simulink model "untitled"  (R2016a)
settings: Solver=VariableStepAuto  StartTime=0.0  StopTime=10.0  RelTol=1e-3
libraries: simulink x1
settings Model: Creator=wojta  LastModifiedBy=wojta

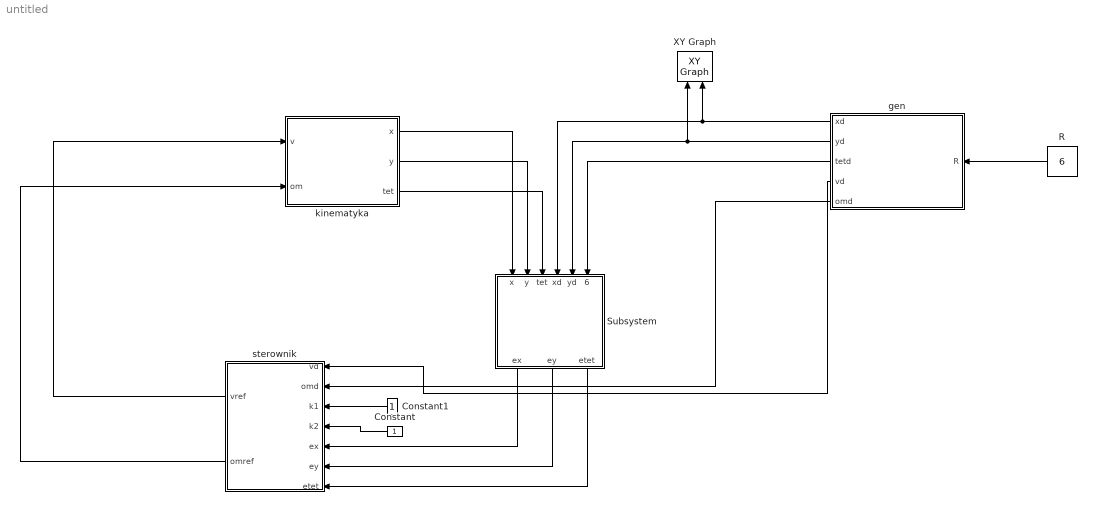
== system untitled ==
  Constant : Constant
  Constant1 : Constant
  R : Constant  Value=6
  Subsystem : Subsystem
  XY Graph : simulink/Sinks/XY Graph  xmin=-6  xmax=6  ymin=-6  ymax=6  st=-1
  gen : Subsystem
  kinematyka : Subsystem
  sterownik : Subsystem
  wires:
  R/1 -> gen/1(R)
  sterownik/1(vref) -> kinematyka/1(v)
  sterownik/2(omref) -> kinematyka/2(om)
  kinematyka/1(x) -> Subsystem/1(x)
  kinematyka/2(y) -> Subsystem/2(y)
  kinematyka/3(tet) -> Subsystem/3(tet)
  gen/1(xd) -> XY Graph/2, Subsystem/4(xd)
  gen/2(yd) -> XY Graph/1, Subsystem/5(yd)
  gen/3(tetd) -> Subsystem/6(tetd)
  Subsystem/1(ex) -> sterownik/5(ex)
  Subsystem/2(ey) -> sterownik/6(ey)
  Subsystem/3(etet) -> sterownik/7(etet)
  gen/4(vd) -> sterownik/1(vd)
  gen/5(omd) -> sterownik/2(omd)
  Constant1/1 -> sterownik/3(k1)
  Constant/1 -> sterownik/4(k2)

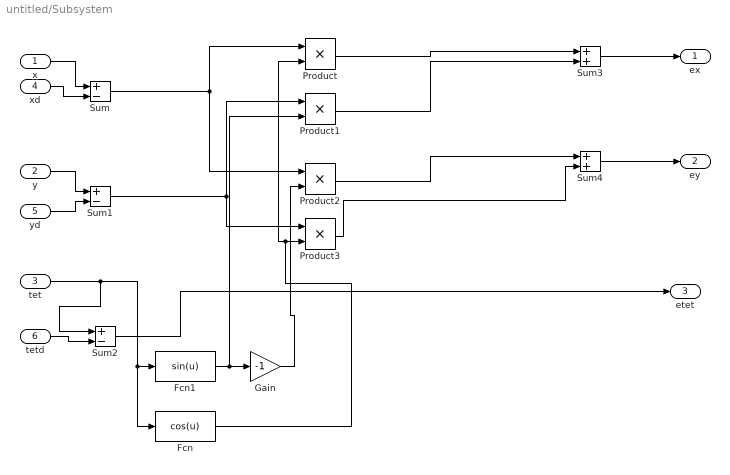
== system untitled/Subsystem ==
  x : Inport
  y : Inport  Port=2
  tet : Inport  Port=3
  xd : Inport  Port=4
  yd : Inport  Port=5
  tetd : Inport  Port=6
  Fcn : Fcn  Expr=cos(u)
  Fcn1 : Fcn  Expr=sin(u)
  Gain : Gain  Gain=-1
  Product{,1..3} (4 alike) : Product
  Sum : Sum  Inputs=+-
  Sum1 : Sum  Inputs=+-
  Sum2 : Sum  Inputs=+-
  Sum3 : Sum
  Sum4 : Sum
  ex : Outport
  ey : Outport  Port=2
  etet : Outport  Port=3
  wires:
  xd/1 -> Sum/2
  yd/1 -> Sum1/2
  Product3/1 -> Sum4/2
  tetd/1 -> Sum2/2
  Fcn1/1 -> Product1/2, Gain/1
  Product1/1 -> Sum3/2
  tet/1 -> Fcn/1, Fcn1/1, Sum2/1
  Gain/1 -> Product2/2
  Product2/1 -> Sum4/1
  Sum2/1 -> etet/1
  y/1 -> Sum1/1
  Product/1 -> Sum3/1
  Sum1/1 -> Product3/1, Product1/1
  Sum4/1 -> ey/1
  x/1 -> Sum/1
  Fcn/1 -> Product/2, Product3/2
  Sum3/1 -> ex/1
  Sum/1 -> Product/1, Product2/1

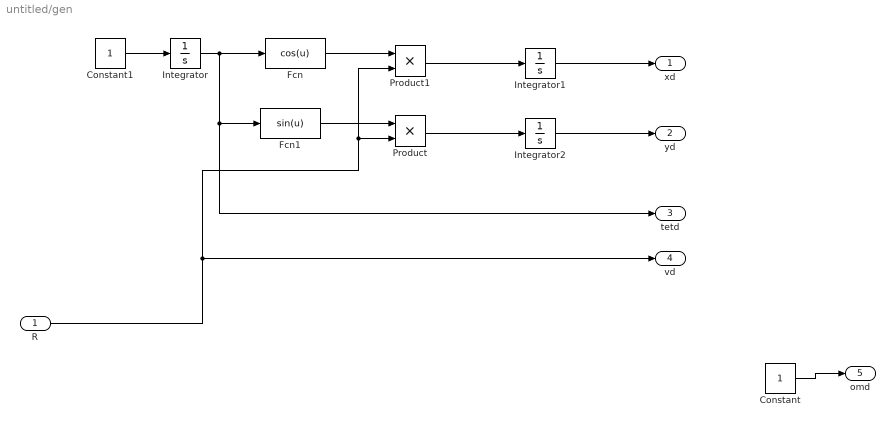
== system untitled/gen ==
  R : Inport
  Constant : Constant
  Constant1 : Constant
  Fcn : Fcn  Expr=cos(u)
  Fcn1 : Fcn  Expr=sin(u)
  Integrator : Integrator
  Integrator1 : Integrator
  Integrator2 : Integrator  InitialCondition=-6
  Product : Product
  Product1 : Product
  xd : Outport
  yd : Outport  Port=2
  tetd : Outport  Port=3
  vd : Outport  Port=4
  omd : Outport  Port=5
  wires:
  Constant/1 -> omd/1
  R/1 -> Product1/2, Product/2, vd/1
  Constant1/1 -> Integrator/1
  Integrator/1 -> Fcn1/1, tetd/1, Fcn/1
  Fcn1/1 -> Product/1
  Fcn/1 -> Product1/1
  Product/1 -> Integrator2/1
  Product1/1 -> Integrator1/1
  Integrator1/1 -> xd/1
  Integrator2/1 -> yd/1

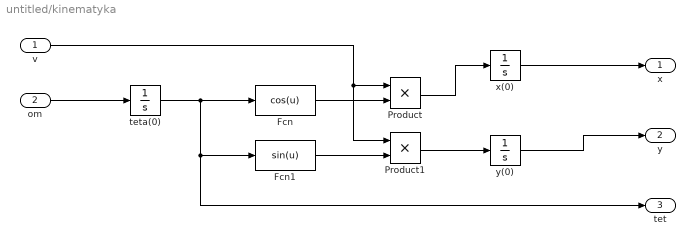
== system untitled/kinematyka ==
  v : Inport
  om : Inport  Port=2
  Fcn : Fcn  Expr=cos(u)
  Fcn1 : Fcn  Expr=sin(u)
  Product : Product
  Product1 : Product
  teta(0) : Integrator
  x(0) : Integrator
  y(0) : Integrator  InitialCondition=-6
  x : Outport
  y : Outport  Port=2
  tet : Outport  Port=3
  wires:
  Fcn1/1 -> Product1/2
  v/1 -> Product1/1, Product/1
  teta(0)/1 -> tet/1, Fcn1/1, Fcn/1
  x(0)/1 -> x/1
  om/1 -> teta(0)/1
  Product1/1 -> y(0)/1
  y(0)/1 -> y/1
  Fcn/1 -> Product/2
  Product/1 -> x(0)/1

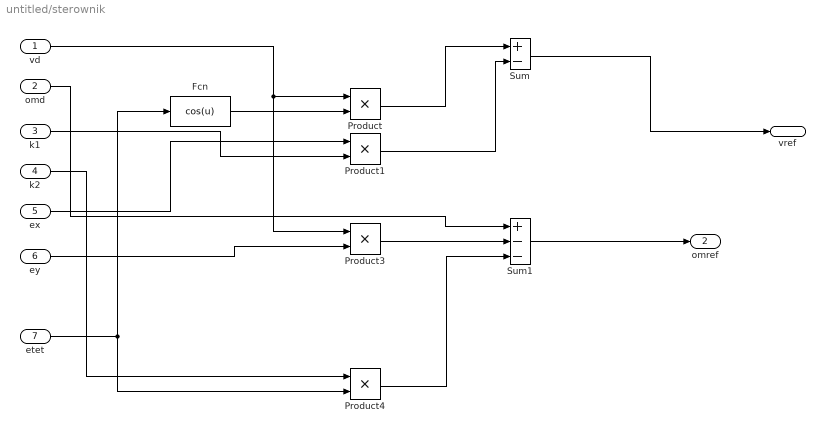
== system untitled/sterownik ==
  vd : Inport
  omd : Inport  Port=2
  k1 : Inport  Port=3
  k2 : Inport  Port=4
  ex : Inport  Port=5
  ey : Inport  Port=6
  etet : Inport  Port=7
  Fcn : Fcn  Expr=cos(u)
  Product{,1,3..4} (4 alike) : Product
  Sum : Sum  Inputs=+-
  Sum1 : Sum  Inputs=+--
  vref : Outport
  omref : Outport  Port=2
  wires:
  ex/1 -> Product1/1
  Product4/1 -> Sum1/3
  Sum1/1 -> omref/1
  k1/1 -> Product1/2
  ey/1 -> Product3/2
  etet/1 -> Fcn/1, Product4/2
  omd/1 -> Sum1/1
  Product3/1 -> Sum1/2
  Fcn/1 -> Product/2
  vd/1 -> Product3/1, Product/1
  k2/1 -> Product4/1
  Sum/1 -> vref/1
  Product1/1 -> Sum/2
  Product/1 -> Sum/1
